simulink model "elevator"  (R2020a)
settings: Solver=VariableStepAuto  StartTime=0.0  StopTime=inf  RelTol=1e-3
PreLoadFcn:
  | slplc.api.loadDataTypes;
undefined symbols (not defined in the file): BOOL, DINT, INT, slplc
libraries: simulink x1
(part 30 of 38)

== system elevator/PLCControllerSuite/__Logic/Task/Program/__Logic/EQU/RungInOverride/ForceRungInFalseRead/__CoreLabelRead ==
  DataRead : DataStoreRead  DataStoreName=x_PLCLabel__s4_3653__Force_RungIn_False
  Out1 : Outport  VectorParamsAs1DForOutWhenUnconnected=off
  wires:
  DataRead/1 -> Out1/1

== system elevator/PLCControllerSuite/__Logic/Task/Program/__Logic/EQU1/RungInOverride/ForceRungInFalseRead/__CoreLabelRead ==
  DataRead : DataStoreRead  DataStoreName=x_PLCLabel__s4_3653__Force_RungIn_False
  Out1 : Outport  VectorParamsAs1DForOutWhenUnconnected=off
  wires:
  DataRead/1 -> Out1/1

== system elevator/PLCControllerSuite/__Logic/Task/Program/__Logic/EQU2/RungInOverride/ForceRungInFalseRead/__CoreLabelRead ==
  DataRead : DataStoreRead  DataStoreName=x_PLCLabel__s4_3653__Force_RungIn_False
  Out1 : Outport  VectorParamsAs1DForOutWhenUnconnected=off
  wires:
  DataRead/1 -> Out1/1

== system elevator/PLCControllerSuite/__Logic/Task/Program/__Logic/EQU3/RungInOverride/ForceRungInFalseRead/__CoreLabelRead ==
  DataRead : DataStoreRead  DataStoreName=x_PLCLabel__s4_3653__Force_RungIn_False
  Out1 : Outport  VectorParamsAs1DForOutWhenUnconnected=off
  wires:
  DataRead/1 -> Out1/1

== system elevator/PLCControllerSuite/__Logic/Task/Program/__Logic/GRT/RungInOverride/ForceRungInFalseRead/__CoreLabelRead ==
  DataRead : DataStoreRead  DataStoreName=x_PLCLabel__s4_3653__Force_RungIn_False
  Out1 : Outport  VectorParamsAs1DForOutWhenUnconnected=off
  wires:
  DataRead/1 -> Out1/1

== system elevator/PLCControllerSuite/__Logic/Task/Program/__Logic/LEQ/RungInOverride/ForceRungInFalseRead/__CoreLabelRead ==
  DataRead : DataStoreRead  DataStoreName=x_PLCLabel__s4_3653__Force_RungIn_False
  Out1 : Outport  VectorParamsAs1DForOutWhenUnconnected=off
  wires:
  DataRead/1 -> Out1/1

== system elevator/PLCControllerSuite/__Logic/Task/Program/__Logic/MOV/RungInOverride/ForceRungInFalseRead/__CoreLabelRead ==
  DataRead : DataStoreRead  DataStoreName=x_PLCLabel__s4_3653__Force_RungIn_False
  Out1 : Outport  VectorParamsAs1DForOutWhenUnconnected=off
  wires:
  DataRead/1 -> Out1/1

== system elevator/PLCControllerSuite/__Logic/Task/Program/__Logic/MOV/RungOutOverride/BlockEnableRead/__CoreLabelRead ==
  DataRead : DataStoreRead  DataStoreName=x_PLCLabel__s4_3653__Block_Enable
  Out1 : Outport  VectorParamsAs1DForOutWhenUnconnected=off
  wires:
  DataRead/1 -> Out1/1

== system elevator/PLCControllerSuite/__Logic/Task/Program/__Logic/MOV/RungOutOverride/VariableWriteEnableWrite/__CoreLabelWrite ==
  In1 : Inport
  DataWrite : DataStoreWrite  DataStoreName=x_PLCLabel__s4_3653__Variable_Write_Enable
  wires:
  In1/1 -> DataWrite/1

== system elevator/PLCControllerSuite/__Logic/Task/Program/__Logic/MOV1/RungInOverride/ForceRungInFalseRead/__CoreLabelRead ==
  DataRead : DataStoreRead  DataStoreName=x_PLCLabel__s4_3653__Force_RungIn_False
  Out1 : Outport  VectorParamsAs1DForOutWhenUnconnected=off
  wires:
  DataRead/1 -> Out1/1

== system elevator/PLCControllerSuite/__Logic/Task/Program/__Logic/MOV1/RungOutOverride/BlockEnableRead/__CoreLabelRead ==
  DataRead : DataStoreRead  DataStoreName=x_PLCLabel__s4_3653__Block_Enable
  Out1 : Outport  VectorParamsAs1DForOutWhenUnconnected=off
  wires:
  DataRead/1 -> Out1/1

== system elevator/PLCControllerSuite/__Logic/Task/Program/__Logic/MOV1/RungOutOverride/VariableWriteEnableWrite/__CoreLabelWrite ==
  In1 : Inport
  DataWrite : DataStoreWrite  DataStoreName=x_PLCLabel__s4_3653__Variable_Write_Enable
  wires:
  In1/1 -> DataWrite/1

== system elevator/PLCControllerSuite/__Logic/Task/Program/__Logic/MOV2/RungInOverride/ForceRungInFalseRead/__CoreLabelRead ==
  DataRead : DataStoreRead  DataStoreName=x_PLCLabel__s4_3653__Force_RungIn_False
  Out1 : Outport  VectorParamsAs1DForOutWhenUnconnected=off
  wires:
  DataRead/1 -> Out1/1

== system elevator/PLCControllerSuite/__Logic/Task/Program/__Logic/MOV2/RungOutOverride/BlockEnableRead/__CoreLabelRead ==
  DataRead : DataStoreRead  DataStoreName=x_PLCLabel__s4_3653__Block_Enable
  Out1 : Outport  VectorParamsAs1DForOutWhenUnconnected=off
  wires:
  DataRead/1 -> Out1/1

== system elevator/PLCControllerSuite/__Logic/Task/Program/__Logic/MOV2/RungOutOverride/VariableWriteEnableWrite/__CoreLabelWrite ==
  In1 : Inport
  DataWrite : DataStoreWrite  DataStoreName=x_PLCLabel__s4_3653__Variable_Write_Enable
  wires:
  In1/1 -> DataWrite/1

== system elevator/PLCControllerSuite/__Logic/Task/Program/__Logic/MOV3/RungInOverride/ForceRungInFalseRead/__CoreLabelRead ==
  DataRead : DataStoreRead  DataStoreName=x_PLCLabel__s4_3653__Force_RungIn_False
  Out1 : Outport  VectorParamsAs1DForOutWhenUnconnected=off
  wires:
  DataRead/1 -> Out1/1

== system elevator/PLCControllerSuite/__Logic/Task/Program/__Logic/MOV3/RungOutOverride/BlockEnableRead/__CoreLabelRead ==
  DataRead : DataStoreRead  DataStoreName=x_PLCLabel__s4_3653__Block_Enable
  Out1 : Outport  VectorParamsAs1DForOutWhenUnconnected=off
  wires:
  DataRead/1 -> Out1/1

== system elevator/PLCControllerSuite/__Logic/Task/Program/__Logic/MOV3/RungOutOverride/VariableWriteEnableWrite/__CoreLabelWrite ==
  In1 : Inport
  DataWrite : DataStoreWrite  DataStoreName=x_PLCLabel__s4_3653__Variable_Write_Enable
  wires:
  In1/1 -> DataWrite/1

== system elevator/PLCControllerSuite/__Logic/Task/Program/__Logic/MOV4/RungInOverride/ForceRungInFalseRead/__CoreLabelRead ==
  DataRead : DataStoreRead  DataStoreName=x_PLCLabel__s4_3653__Force_RungIn_False
  Out1 : Outport  VectorParamsAs1DForOutWhenUnconnected=off
  wires:
  DataRead/1 -> Out1/1

== system elevator/PLCControllerSuite/__Logic/Task/Program/__Logic/MOV4/RungOutOverride/BlockEnableRead/__CoreLabelRead ==
  DataRead : DataStoreRead  DataStoreName=x_PLCLabel__s4_3653__Block_Enable
  Out1 : Outport  VectorParamsAs1DForOutWhenUnconnected=off
  wires:
  DataRead/1 -> Out1/1

== system elevator/PLCControllerSuite/__Logic/Task/Program/__Logic/MOV4/RungOutOverride/VariableWriteEnableWrite/__CoreLabelWrite ==
  In1 : Inport
  DataWrite : DataStoreWrite  DataStoreName=x_PLCLabel__s4_3653__Variable_Write_Enable
  wires:
  In1/1 -> DataWrite/1

== system elevator/PLCControllerSuite/__Logic/Task/Program/__Logic/MUL/RungInOverride/ForceRungInFalseRead/__CoreLabelRead ==
  DataRead : DataStoreRead  DataStoreName=x_PLCLabel__s4_3653__Force_RungIn_False
  Out1 : Outport  VectorParamsAs1DForOutWhenUnconnected=off
  wires:
  DataRead/1 -> Out1/1

== system elevator/PLCControllerSuite/__Logic/Task/Program/__Logic/MUL/RungOutOverride/BlockEnableRead/__CoreLabelRead ==
  DataRead : DataStoreRead  DataStoreName=x_PLCLabel__s4_3653__Block_Enable
  Out1 : Outport  VectorParamsAs1DForOutWhenUnconnected=off
  wires:
  DataRead/1 -> Out1/1

== system elevator/PLCControllerSuite/__Logic/Task/Program/__Logic/MUL/RungOutOverride/VariableWriteEnableWrite/__CoreLabelWrite ==
  In1 : Inport
  DataWrite : DataStoreWrite  DataStoreName=x_PLCLabel__s4_3653__Variable_Write_Enable
  wires:
  In1/1 -> DataWrite/1

== system elevator/PLCControllerSuite/__Logic/Task/Program/__Logic/OTE/Instruction_Enable/Initialize Function/__CoreVarWrite ==
  u : Inport
  DataWrite : DataStoreWrite  DataStoreName=xxx_PLC_VAR_StartHold
  wires:
  u/1 -> DataWrite/1

== system elevator/PLCControllerSuite/__Logic/Task/Program/__Logic/OTE/Instruction_Enable/Rung-condition is false/__CoreVarWrite ==
  u : Inport
  DataWrite : DataStoreWrite  DataStoreName=xxx_PLC_VAR_StartHold
  wires:
  u/1 -> DataWrite/1

== system elevator/PLCControllerSuite/__Logic/Task/Program/__Logic/OTE/Instruction_Enable/Rung-condition-in is true/__CoreVarWrite ==
  u : Inport
  DataWrite : DataStoreWrite  DataStoreName=xxx_PLC_VAR_StartHold
  wires:
  u/1 -> DataWrite/1

== system elevator/PLCControllerSuite/__Logic/Task/Program/__Logic/OTE/RungInOverride/ForceRungInFalseRead/__CoreLabelRead ==
  DataRead : DataStoreRead  DataStoreName=x_PLCLabel__s4_3653__Force_RungIn_False
  Out1 : Outport  VectorParamsAs1DForOutWhenUnconnected=off
  wires:
  DataRead/1 -> Out1/1

== system elevator/PLCControllerSuite/__Logic/Task/Program/__Logic/OTE1/Instruction_Enable/Initialize Function/__CoreVarWrite ==
  u : Inport
  DataWrite : DataStoreWrite  DataStoreName=xxx_PLC_VAR_F1PBHold
  wires:
  u/1 -> DataWrite/1

== system elevator/PLCControllerSuite/__Logic/Task/Program/__Logic/OTE1/Instruction_Enable/Rung-condition is false/__CoreVarWrite ==
  u : Inport
  DataWrite : DataStoreWrite  DataStoreName=xxx_PLC_VAR_F1PBHold
  wires:
  u/1 -> DataWrite/1

== system elevator/PLCControllerSuite/__Logic/Task/Program/__Logic/OTE1/Instruction_Enable/Rung-condition-in is true/__CoreVarWrite ==
  u : Inport
  DataWrite : DataStoreWrite  DataStoreName=xxx_PLC_VAR_F1PBHold
  wires:
  u/1 -> DataWrite/1

== system elevator/PLCControllerSuite/__Logic/Task/Program/__Logic/OTE1/RungInOverride/ForceRungInFalseRead/__CoreLabelRead ==
  DataRead : DataStoreRead  DataStoreName=x_PLCLabel__s4_3653__Force_RungIn_False
  Out1 : Outport  VectorParamsAs1DForOutWhenUnconnected=off
  wires:
  DataRead/1 -> Out1/1

== system elevator/PLCControllerSuite/__Logic/Task/Program/__Logic/OTE10/Instruction_Enable/Initialize Function/__CoreVarWrite ==
  u : Inport
  DataWrite : DataStoreWrite  DataStoreName=xxx_PLC_VAR_MemoryGoDown
  wires:
  u/1 -> DataWrite/1

== system elevator/PLCControllerSuite/__Logic/Task/Program/__Logic/OTE10/Instruction_Enable/Rung-condition is false/__CoreVarWrite ==
  u : Inport
  DataWrite : DataStoreWrite  DataStoreName=xxx_PLC_VAR_MemoryGoDown
  wires:
  u/1 -> DataWrite/1

== system elevator/PLCControllerSuite/__Logic/Task/Program/__Logic/OTE10/Instruction_Enable/Rung-condition-in is true/__CoreVarWrite ==
  u : Inport
  DataWrite : DataStoreWrite  DataStoreName=xxx_PLC_VAR_MemoryGoDown
  wires:
  u/1 -> DataWrite/1

== system elevator/PLCControllerSuite/__Logic/Task/Program/__Logic/OTE10/RungInOverride/ForceRungInFalseRead/__CoreLabelRead ==
  DataRead : DataStoreRead  DataStoreName=x_PLCLabel__s4_3653__Force_RungIn_False
  Out1 : Outport  VectorParamsAs1DForOutWhenUnconnected=off
  wires:
  DataRead/1 -> Out1/1

== system elevator/PLCControllerSuite/__Logic/Task/Program/__Logic/OTE11/Instruction_Enable/Initialize Function/__CoreVarWrite ==
  u : Inport
  DataWrite : DataStoreWrite  DataStoreName=xxx_PLC_VAR_RMPUPTRG
  wires:
  u/1 -> DataWrite/1

== system elevator/PLCControllerSuite/__Logic/Task/Program/__Logic/OTE11/Instruction_Enable/Rung-condition is false/__CoreVarWrite ==
  u : Inport
  DataWrite : DataStoreWrite  DataStoreName=xxx_PLC_VAR_RMPUPTRG
  wires:
  u/1 -> DataWrite/1

== system elevator/PLCControllerSuite/__Logic/Task/Program/__Logic/OTE11/Instruction_Enable/Rung-condition-in is true/__CoreVarWrite ==
  u : Inport
  DataWrite : DataStoreWrite  DataStoreName=xxx_PLC_VAR_RMPUPTRG
  wires:
  u/1 -> DataWrite/1

== system elevator/PLCControllerSuite/__Logic/Task/Program/__Logic/OTE11/RungInOverride/ForceRungInFalseRead/__CoreLabelRead ==
  DataRead : DataStoreRead  DataStoreName=x_PLCLabel__s4_3653__Force_RungIn_False
  Out1 : Outport  VectorParamsAs1DForOutWhenUnconnected=off
  wires:
  DataRead/1 -> Out1/1

== system elevator/PLCControllerSuite/__Logic/Task/Program/__Logic/OTE12/Instruction_Enable/Initialize Function/__CoreVarWrite ==
  u : Inport
  DataWrite : DataStoreWrite  DataStoreName=xxx_PLC_VAR_RMPUP
  wires:
  u/1 -> DataWrite/1

== system elevator/PLCControllerSuite/__Logic/Task/Program/__Logic/OTE12/Instruction_Enable/Rung-condition is false/__CoreVarWrite ==
  u : Inport
  DataWrite : DataStoreWrite  DataStoreName=xxx_PLC_VAR_RMPUP
  wires:
  u/1 -> DataWrite/1

== system elevator/PLCControllerSuite/__Logic/Task/Program/__Logic/OTE12/Instruction_Enable/Rung-condition-in is true/__CoreVarWrite ==
  u : Inport
  DataWrite : DataStoreWrite  DataStoreName=xxx_PLC_VAR_RMPUP
  wires:
  u/1 -> DataWrite/1

== system elevator/PLCControllerSuite/__Logic/Task/Program/__Logic/OTE12/RungInOverride/ForceRungInFalseRead/__CoreLabelRead ==
  DataRead : DataStoreRead  DataStoreName=x_PLCLabel__s4_3653__Force_RungIn_False
  Out1 : Outport  VectorParamsAs1DForOutWhenUnconnected=off
  wires:
  DataRead/1 -> Out1/1

== system elevator/PLCControllerSuite/__Logic/Task/Program/__Logic/OTE13/Instruction_Enable/Initialize Function/__CoreVarWrite ==
  u : Inport
  DataWrite : DataStoreWrite  DataStoreName=xxx_PLC_VAR_RMPDN
  wires:
  u/1 -> DataWrite/1

== system elevator/PLCControllerSuite/__Logic/Task/Program/__Logic/OTE13/Instruction_Enable/Rung-condition is false/__CoreVarWrite ==
  u : Inport
  DataWrite : DataStoreWrite  DataStoreName=xxx_PLC_VAR_RMPDN
  wires:
  u/1 -> DataWrite/1

== system elevator/PLCControllerSuite/__Logic/Task/Program/__Logic/OTE13/Instruction_Enable/Rung-condition-in is true/__CoreVarWrite ==
  u : Inport
  DataWrite : DataStoreWrite  DataStoreName=xxx_PLC_VAR_RMPDN
  wires:
  u/1 -> DataWrite/1

== system elevator/PLCControllerSuite/__Logic/Task/Program/__Logic/OTE13/RungInOverride/ForceRungInFalseRead/__CoreLabelRead ==
  DataRead : DataStoreRead  DataStoreName=x_PLCLabel__s4_3653__Force_RungIn_False
  Out1 : Outport  VectorParamsAs1DForOutWhenUnconnected=off
  wires:
  DataRead/1 -> Out1/1

== system elevator/PLCControllerSuite/__Logic/Task/Program/__Logic/OTE14/Instruction_Enable/Initialize Function/__CoreVarWrite ==
  u : Inport
  DataWrite : DataStoreWrite  DataStoreName=xxx_PLC_VAR_RMPUPKIL
  wires:
  u/1 -> DataWrite/1

== system elevator/PLCControllerSuite/__Logic/Task/Program/__Logic/OTE14/Instruction_Enable/Rung-condition is false/__CoreVarWrite ==
  u : Inport
  DataWrite : DataStoreWrite  DataStoreName=xxx_PLC_VAR_RMPUPKIL
  wires:
  u/1 -> DataWrite/1

== system elevator/PLCControllerSuite/__Logic/Task/Program/__Logic/OTE14/Instruction_Enable/Rung-condition-in is true/__CoreVarWrite ==
  u : Inport
  DataWrite : DataStoreWrite  DataStoreName=xxx_PLC_VAR_RMPUPKIL
  wires:
  u/1 -> DataWrite/1

== system elevator/PLCControllerSuite/__Logic/Task/Program/__Logic/OTE14/RungInOverride/ForceRungInFalseRead/__CoreLabelRead ==
  DataRead : DataStoreRead  DataStoreName=x_PLCLabel__s4_3653__Force_RungIn_False
  Out1 : Outport  VectorParamsAs1DForOutWhenUnconnected=off
  wires:
  DataRead/1 -> Out1/1

== system elevator/PLCControllerSuite/__Logic/Task/Program/__Logic/OTE15/Instruction_Enable/Initialize Function/__CoreVarWrite ==
  u : Inport
  DataWrite : DataStoreWrite  DataStoreName=xxx_PLC_VAR_TempS1HUp
  wires:
  u/1 -> DataWrite/1

== system elevator/PLCControllerSuite/__Logic/Task/Program/__Logic/OTE15/Instruction_Enable/Rung-condition is false/__CoreVarWrite ==
  u : Inport
  DataWrite : DataStoreWrite  DataStoreName=xxx_PLC_VAR_TempS1HUp
  wires:
  u/1 -> DataWrite/1

== system elevator/PLCControllerSuite/__Logic/Task/Program/__Logic/OTE15/Instruction_Enable/Rung-condition-in is true/__CoreVarWrite ==
  u : Inport
  DataWrite : DataStoreWrite  DataStoreName=xxx_PLC_VAR_TempS1HUp
  wires:
  u/1 -> DataWrite/1

== system elevator/PLCControllerSuite/__Logic/Task/Program/__Logic/OTE15/RungInOverride/ForceRungInFalseRead/__CoreLabelRead ==
  DataRead : DataStoreRead  DataStoreName=x_PLCLabel__s4_3653__Force_RungIn_False
  Out1 : Outport  VectorParamsAs1DForOutWhenUnconnected=off
  wires:
  DataRead/1 -> Out1/1

== system elevator/PLCControllerSuite/__Logic/Task/Program/__Logic/OTE16/Instruction_Enable/Initialize Function/__CoreVarWrite ==
  u : Inport
  DataWrite : DataStoreWrite  DataStoreName=xxx_PLC_VAR_TempS2LUp
  wires:
  u/1 -> DataWrite/1

== system elevator/PLCControllerSuite/__Logic/Task/Program/__Logic/OTE16/Instruction_Enable/Rung-condition is false/__CoreVarWrite ==
  u : Inport
  DataWrite : DataStoreWrite  DataStoreName=xxx_PLC_VAR_TempS2LUp
  wires:
  u/1 -> DataWrite/1

== system elevator/PLCControllerSuite/__Logic/Task/Program/__Logic/OTE16/Instruction_Enable/Rung-condition-in is true/__CoreVarWrite ==
  u : Inport
  DataWrite : DataStoreWrite  DataStoreName=xxx_PLC_VAR_TempS2LUp
  wires:
  u/1 -> DataWrite/1

== system elevator/PLCControllerSuite/__Logic/Task/Program/__Logic/OTE16/RungInOverride/ForceRungInFalseRead/__CoreLabelRead ==
  DataRead : DataStoreRead  DataStoreName=x_PLCLabel__s4_3653__Force_RungIn_False
  Out1 : Outport  VectorParamsAs1DForOutWhenUnconnected=off
  wires:
  DataRead/1 -> Out1/1

== system elevator/PLCControllerSuite/__Logic/Task/Program/__Logic/OTE17/Instruction_Enable/Initialize Function/__CoreVarWrite ==
  u : Inport
  DataWrite : DataStoreWrite  DataStoreName=xxx_PLC_VAR_TempS3LUp
  wires:
  u/1 -> DataWrite/1

== system elevator/PLCControllerSuite/__Logic/Task/Program/__Logic/OTE17/Instruction_Enable/Rung-condition is false/__CoreVarWrite ==
  u : Inport
  DataWrite : DataStoreWrite  DataStoreName=xxx_PLC_VAR_TempS3LUp
  wires:
  u/1 -> DataWrite/1

== system elevator/PLCControllerSuite/__Logic/Task/Program/__Logic/OTE17/Instruction_Enable/Rung-condition-in is true/__CoreVarWrite ==
  u : Inport
  DataWrite : DataStoreWrite  DataStoreName=xxx_PLC_VAR_TempS3LUp
  wires:
  u/1 -> DataWrite/1

== system elevator/PLCControllerSuite/__Logic/Task/Program/__Logic/OTE17/RungInOverride/ForceRungInFalseRead/__CoreLabelRead ==
  DataRead : DataStoreRead  DataStoreName=x_PLCLabel__s4_3653__Force_RungIn_False
  Out1 : Outport  VectorParamsAs1DForOutWhenUnconnected=off
  wires:
  DataRead/1 -> Out1/1

== system elevator/PLCControllerSuite/__Logic/Task/Program/__Logic/OTE18/Instruction_Enable/Initialize Function/__CoreVarWrite ==
  u : Inport
  DataWrite : DataStoreWrite  DataStoreName=xxx_PLC_VAR_TempS2HDown
  wires:
  u/1 -> DataWrite/1

== system elevator/PLCControllerSuite/__Logic/Task/Program/__Logic/OTE18/Instruction_Enable/Rung-condition is false/__CoreVarWrite ==
  u : Inport
  DataWrite : DataStoreWrite  DataStoreName=xxx_PLC_VAR_TempS2HDown
  wires:
  u/1 -> DataWrite/1

== system elevator/PLCControllerSuite/__Logic/Task/Program/__Logic/OTE18/Instruction_Enable/Rung-condition-in is true/__CoreVarWrite ==
  u : Inport
  DataWrite : DataStoreWrite  DataStoreName=xxx_PLC_VAR_TempS2HDown
  wires:
  u/1 -> DataWrite/1

== system elevator/PLCControllerSuite/__Logic/Task/Program/__Logic/OTE18/RungInOverride/ForceRungInFalseRead/__CoreLabelRead ==
  DataRead : DataStoreRead  DataStoreName=x_PLCLabel__s4_3653__Force_RungIn_False
  Out1 : Outport  VectorParamsAs1DForOutWhenUnconnected=off
  wires:
  DataRead/1 -> Out1/1

== system elevator/PLCControllerSuite/__Logic/Task/Program/__Logic/OTE19/Instruction_Enable/Initialize Function/__CoreVarWrite ==
  u : Inport
  DataWrite : DataStoreWrite  DataStoreName=xxx_PLC_VAR_TempS2LDown
  wires:
  u/1 -> DataWrite/1

== system elevator/PLCControllerSuite/__Logic/Task/Program/__Logic/OTE19/Instruction_Enable/Rung-condition is false/__CoreVarWrite ==
  u : Inport
  DataWrite : DataStoreWrite  DataStoreName=xxx_PLC_VAR_TempS2LDown
  wires:
  u/1 -> DataWrite/1

== system elevator/PLCControllerSuite/__Logic/Task/Program/__Logic/OTE19/Instruction_Enable/Rung-condition-in is true/__CoreVarWrite ==
  u : Inport
  DataWrite : DataStoreWrite  DataStoreName=xxx_PLC_VAR_TempS2LDown
  wires:
  u/1 -> DataWrite/1

== system elevator/PLCControllerSuite/__Logic/Task/Program/__Logic/OTE19/RungInOverride/ForceRungInFalseRead/__CoreLabelRead ==
  DataRead : DataStoreRead  DataStoreName=x_PLCLabel__s4_3653__Force_RungIn_False
  Out1 : Outport  VectorParamsAs1DForOutWhenUnconnected=off
  wires:
  DataRead/1 -> Out1/1

== system elevator/PLCControllerSuite/__Logic/Task/Program/__Logic/OTE2/Instruction_Enable/Initialize Function/__CoreVarWrite ==
  u : Inport
  DataWrite : DataStoreWrite  DataStoreName=xxx_PLC_VAR_F2PBHold
  wires:
  u/1 -> DataWrite/1

== system elevator/PLCControllerSuite/__Logic/Task/Program/__Logic/OTE2/Instruction_Enable/Rung-condition is false/__CoreVarWrite ==
  u : Inport
  DataWrite : DataStoreWrite  DataStoreName=xxx_PLC_VAR_F2PBHold
  wires:
  u/1 -> DataWrite/1

== system elevator/PLCControllerSuite/__Logic/Task/Program/__Logic/OTE2/Instruction_Enable/Rung-condition-in is true/__CoreVarWrite ==
  u : Inport
  DataWrite : DataStoreWrite  DataStoreName=xxx_PLC_VAR_F2PBHold
  wires:
  u/1 -> DataWrite/1

== system elevator/PLCControllerSuite/__Logic/Task/Program/__Logic/OTE2/RungInOverride/ForceRungInFalseRead/__CoreLabelRead ==
  DataRead : DataStoreRead  DataStoreName=x_PLCLabel__s4_3653__Force_RungIn_False
  Out1 : Outport  VectorParamsAs1DForOutWhenUnconnected=off
  wires:
  DataRead/1 -> Out1/1

== system elevator/PLCControllerSuite/__Logic/Task/Program/__Logic/OTE20/Instruction_Enable/Initialize Function/__CoreVarWrite ==
  u : Inport
  DataWrite : DataStoreWrite  DataStoreName=xxx_PLC_VAR_TempS1HDown
  wires:
  u/1 -> DataWrite/1

== system elevator/PLCControllerSuite/__Logic/Task/Program/__Logic/OTE20/Instruction_Enable/Rung-condition is false/__CoreVarWrite ==
  u : Inport
  DataWrite : DataStoreWrite  DataStoreName=xxx_PLC_VAR_TempS1HDown
  wires:
  u/1 -> DataWrite/1

== system elevator/PLCControllerSuite/__Logic/Task/Program/__Logic/OTE20/Instruction_Enable/Rung-condition-in is true/__CoreVarWrite ==
  u : Inport
  DataWrite : DataStoreWrite  DataStoreName=xxx_PLC_VAR_TempS1HDown
  wires:
  u/1 -> DataWrite/1

== system elevator/PLCControllerSuite/__Logic/Task/Program/__Logic/OTE20/RungInOverride/ForceRungInFalseRead/__CoreLabelRead ==
  DataRead : DataStoreRead  DataStoreName=x_PLCLabel__s4_3653__Force_RungIn_False
  Out1 : Outport  VectorParamsAs1DForOutWhenUnconnected=off
  wires:
  DataRead/1 -> Out1/1

== system elevator/PLCControllerSuite/__Logic/Task/Program/__Logic/OTE21/Instruction_Enable/Initialize Function/__CoreVarWrite ==
  u : Inport
  DataWrite : DataStoreWrite  DataStoreName=xxx_PLC_VAR_TempS2HUp
  wires:
  u/1 -> DataWrite/1

== system elevator/PLCControllerSuite/__Logic/Task/Program/__Logic/OTE21/Instruction_Enable/Rung-condition is false/__CoreVarWrite ==
  u : Inport
  DataWrite : DataStoreWrite  DataStoreName=xxx_PLC_VAR_TempS2HUp
  wires:
  u/1 -> DataWrite/1

== system elevator/PLCControllerSuite/__Logic/Task/Program/__Logic/OTE21/Instruction_Enable/Rung-condition-in is true/__CoreVarWrite ==
  u : Inport
  DataWrite : DataStoreWrite  DataStoreName=xxx_PLC_VAR_TempS2HUp
  wires:
  u/1 -> DataWrite/1

== system elevator/PLCControllerSuite/__Logic/Task/Program/__Logic/OTE21/RungInOverride/ForceRungInFalseRead/__CoreLabelRead ==
  DataRead : DataStoreRead  DataStoreName=x_PLCLabel__s4_3653__Force_RungIn_False
  Out1 : Outport  VectorParamsAs1DForOutWhenUnconnected=off
  wires:
  DataRead/1 -> Out1/1

== system elevator/PLCControllerSuite/__Logic/Task/Program/__Logic/OTE22/Instruction_Enable/Initialize Function/__CoreVarWrite ==
  u : Inport
  DataWrite : DataStoreWrite  DataStoreName=xxx_PLC_VAR_TempS3LDown
  wires:
  u/1 -> DataWrite/1

== system elevator/PLCControllerSuite/__Logic/Task/Program/__Logic/OTE22/Instruction_Enable/Rung-condition is false/__CoreVarWrite ==
  u : Inport
  DataWrite : DataStoreWrite  DataStoreName=xxx_PLC_VAR_TempS3LDown
  wires:
  u/1 -> DataWrite/1

== system elevator/PLCControllerSuite/__Logic/Task/Program/__Logic/OTE22/Instruction_Enable/Rung-condition-in is true/__CoreVarWrite ==
  u : Inport
  DataWrite : DataStoreWrite  DataStoreName=xxx_PLC_VAR_TempS3LDown
  wires:
  u/1 -> DataWrite/1

== system elevator/PLCControllerSuite/__Logic/Task/Program/__Logic/OTE22/RungInOverride/ForceRungInFalseRead/__CoreLabelRead ==
  DataRead : DataStoreRead  DataStoreName=x_PLCLabel__s4_3653__Force_RungIn_False
  Out1 : Outport  VectorParamsAs1DForOutWhenUnconnected=off
  wires:
  DataRead/1 -> Out1/1

== system elevator/PLCControllerSuite/__Logic/Task/Program/__Logic/OTE23/Instruction_Enable/Initialize Function/__CoreVarWrite ==
  u : Inport
  DataWrite : DataStoreWrite  DataStoreName=xxx_PLC_VAR_AtFloor1
  wires:
  u/1 -> DataWrite/1

== system elevator/PLCControllerSuite/__Logic/Task/Program/__Logic/OTE23/Instruction_Enable/Rung-condition is false/__CoreVarWrite ==
  u : Inport
  DataWrite : DataStoreWrite  DataStoreName=xxx_PLC_VAR_AtFloor1
  wires:
  u/1 -> DataWrite/1

== system elevator/PLCControllerSuite/__Logic/Task/Program/__Logic/OTE23/Instruction_Enable/Rung-condition-in is true/__CoreVarWrite ==
  u : Inport
  DataWrite : DataStoreWrite  DataStoreName=xxx_PLC_VAR_AtFloor1
  wires:
  u/1 -> DataWrite/1

== system elevator/PLCControllerSuite/__Logic/Task/Program/__Logic/OTE23/RungInOverride/ForceRungInFalseRead/__CoreLabelRead ==
  DataRead : DataStoreRead  DataStoreName=x_PLCLabel__s4_3653__Force_RungIn_False
  Out1 : Outport  VectorParamsAs1DForOutWhenUnconnected=off
  wires:
  DataRead/1 -> Out1/1

== system elevator/PLCControllerSuite/__Logic/Task/Program/__Logic/OTE24/Instruction_Enable/Initialize Function/__CoreVarWrite ==
  u : Inport
  DataWrite : DataStoreWrite  DataStoreName=xxx_PLC_VAR_AtFloor2
  wires:
  u/1 -> DataWrite/1

== system elevator/PLCControllerSuite/__Logic/Task/Program/__Logic/OTE24/Instruction_Enable/Rung-condition is false/__CoreVarWrite ==
  u : Inport
  DataWrite : DataStoreWrite  DataStoreName=xxx_PLC_VAR_AtFloor2
  wires:
  u/1 -> DataWrite/1

== system elevator/PLCControllerSuite/__Logic/Task/Program/__Logic/OTE24/Instruction_Enable/Rung-condition-in is true/__CoreVarWrite ==
  u : Inport
  DataWrite : DataStoreWrite  DataStoreName=xxx_PLC_VAR_AtFloor2
  wires:
  u/1 -> DataWrite/1

== system elevator/PLCControllerSuite/__Logic/Task/Program/__Logic/OTE24/RungInOverride/ForceRungInFalseRead/__CoreLabelRead ==
  DataRead : DataStoreRead  DataStoreName=x_PLCLabel__s4_3653__Force_RungIn_False
  Out1 : Outport  VectorParamsAs1DForOutWhenUnconnected=off
  wires:
  DataRead/1 -> Out1/1

== system elevator/PLCControllerSuite/__Logic/Task/Program/__Logic/OTE25/Instruction_Enable/Initialize Function/__CoreVarWrite ==
  u : Inport
  DataWrite : DataStoreWrite  DataStoreName=xxx_PLC_VAR_AtFloor3
  wires:
  u/1 -> DataWrite/1

== system elevator/PLCControllerSuite/__Logic/Task/Program/__Logic/OTE25/Instruction_Enable/Rung-condition is false/__CoreVarWrite ==
  u : Inport
  DataWrite : DataStoreWrite  DataStoreName=xxx_PLC_VAR_AtFloor3
  wires:
  u/1 -> DataWrite/1

== system elevator/PLCControllerSuite/__Logic/Task/Program/__Logic/OTE25/Instruction_Enable/Rung-condition-in is true/__CoreVarWrite ==
  u : Inport
  DataWrite : DataStoreWrite  DataStoreName=xxx_PLC_VAR_AtFloor3
  wires:
  u/1 -> DataWrite/1

== system elevator/PLCControllerSuite/__Logic/Task/Program/__Logic/OTE25/RungInOverride/ForceRungInFalseRead/__CoreLabelRead ==
  DataRead : DataStoreRead  DataStoreName=x_PLCLabel__s4_3653__Force_RungIn_False
  Out1 : Outport  VectorParamsAs1DForOutWhenUnconnected=off
  wires:
  DataRead/1 -> Out1/1

== system elevator/PLCControllerSuite/__Logic/Task/Program/__Logic/OTE26/Instruction_Enable/Initialize Function/__CoreVarWrite ==
  u : Inport
  DataWrite : DataStoreWrite  DataStoreName=xxx_PLC_VAR_GOINGUP
  wires:
  u/1 -> DataWrite/1

== system elevator/PLCControllerSuite/__Logic/Task/Program/__Logic/OTE26/Instruction_Enable/Rung-condition is false/__CoreVarWrite ==
  u : Inport
  DataWrite : DataStoreWrite  DataStoreName=xxx_PLC_VAR_GOINGUP
  wires:
  u/1 -> DataWrite/1

== system elevator/PLCControllerSuite/__Logic/Task/Program/__Logic/OTE26/Instruction_Enable/Rung-condition-in is true/__CoreVarWrite ==
  u : Inport
  DataWrite : DataStoreWrite  DataStoreName=xxx_PLC_VAR_GOINGUP
  wires:
  u/1 -> DataWrite/1

== system elevator/PLCControllerSuite/__Logic/Task/Program/__Logic/OTE26/RungInOverride/ForceRungInFalseRead/__CoreLabelRead ==
  DataRead : DataStoreRead  DataStoreName=x_PLCLabel__s4_3653__Force_RungIn_False
  Out1 : Outport  VectorParamsAs1DForOutWhenUnconnected=off
  wires:
  DataRead/1 -> Out1/1

== system elevator/PLCControllerSuite/__Logic/Task/Program/__Logic/OTE27/Instruction_Enable/Initialize Function/__CoreVarWrite ==
  u : Inport
  DataWrite : DataStoreWrite  DataStoreName=xxx_PLC_VAR_GOINGDN
  wires:
  u/1 -> DataWrite/1

== system elevator/PLCControllerSuite/__Logic/Task/Program/__Logic/OTE27/Instruction_Enable/Rung-condition is false/__CoreVarWrite ==
  u : Inport
  DataWrite : DataStoreWrite  DataStoreName=xxx_PLC_VAR_GOINGDN
  wires:
  u/1 -> DataWrite/1

== system elevator/PLCControllerSuite/__Logic/Task/Program/__Logic/OTE27/Instruction_Enable/Rung-condition-in is true/__CoreVarWrite ==
  u : Inport
  DataWrite : DataStoreWrite  DataStoreName=xxx_PLC_VAR_GOINGDN
  wires:
  u/1 -> DataWrite/1

== system elevator/PLCControllerSuite/__Logic/Task/Program/__Logic/OTE27/RungInOverride/ForceRungInFalseRead/__CoreLabelRead ==
  DataRead : DataStoreRead  DataStoreName=x_PLCLabel__s4_3653__Force_RungIn_False
  Out1 : Outport  VectorParamsAs1DForOutWhenUnconnected=off
  wires:
  DataRead/1 -> Out1/1

== system elevator/PLCControllerSuite/__Logic/Task/Program/__Logic/OTE28/Instruction_Enable/Initialize Function/__CoreVarWrite ==
  u : Inport
  DataWrite : DataStoreWrite  DataStoreName=xxx_PLC_VAR_MTRON
  wires:
  u/1 -> DataWrite/1

== system elevator/PLCControllerSuite/__Logic/Task/Program/__Logic/OTE28/Instruction_Enable/Rung-condition is false/__CoreVarWrite ==
  u : Inport
  DataWrite : DataStoreWrite  DataStoreName=xxx_PLC_VAR_MTRON
  wires:
  u/1 -> DataWrite/1

== system elevator/PLCControllerSuite/__Logic/Task/Program/__Logic/OTE28/Instruction_Enable/Rung-condition-in is true/__CoreVarWrite ==
  u : Inport
  DataWrite : DataStoreWrite  DataStoreName=xxx_PLC_VAR_MTRON
  wires:
  u/1 -> DataWrite/1

== system elevator/PLCControllerSuite/__Logic/Task/Program/__Logic/OTE28/RungInOverride/ForceRungInFalseRead/__CoreLabelRead ==
  DataRead : DataStoreRead  DataStoreName=x_PLCLabel__s4_3653__Force_RungIn_False
  Out1 : Outport  VectorParamsAs1DForOutWhenUnconnected=off
  wires:
  DataRead/1 -> Out1/1

== system elevator/PLCControllerSuite/__Logic/Task/Program/__Logic/OTE29/Instruction_Enable/Initialize Function/__CoreVarWrite ==
  u : Inport
  DataWrite : DataStoreWrite  DataStoreName=xxx_PLC_VAR_RMPDNTRG
  wires:
  u/1 -> DataWrite/1

== system elevator/PLCControllerSuite/__Logic/Task/Program/__Logic/OTE29/Instruction_Enable/Rung-condition is false/__CoreVarWrite ==
  u : Inport
  DataWrite : DataStoreWrite  DataStoreName=xxx_PLC_VAR_RMPDNTRG
  wires:
  u/1 -> DataWrite/1

== system elevator/PLCControllerSuite/__Logic/Task/Program/__Logic/OTE29/Instruction_Enable/Rung-condition-in is true/__CoreVarWrite ==
  u : Inport
  DataWrite : DataStoreWrite  DataStoreName=xxx_PLC_VAR_RMPDNTRG
  wires:
  u/1 -> DataWrite/1

== system elevator/PLCControllerSuite/__Logic/Task/Program/__Logic/OTE29/RungInOverride/ForceRungInFalseRead/__CoreLabelRead ==
  DataRead : DataStoreRead  DataStoreName=x_PLCLabel__s4_3653__Force_RungIn_False
  Out1 : Outport  VectorParamsAs1DForOutWhenUnconnected=off
  wires:
  DataRead/1 -> Out1/1

== system elevator/PLCControllerSuite/__Logic/Task/Program/__Logic/OTE3/Instruction_Enable/Initialize Function/__CoreVarWrite ==
  u : Inport
  DataWrite : DataStoreWrite  DataStoreName=xxx_PLC_VAR_F3PBHold
  wires:
  u/1 -> DataWrite/1

== system elevator/PLCControllerSuite/__Logic/Task/Program/__Logic/OTE3/Instruction_Enable/Rung-condition is false/__CoreVarWrite ==
  u : Inport
  DataWrite : DataStoreWrite  DataStoreName=xxx_PLC_VAR_F3PBHold
  wires:
  u/1 -> DataWrite/1

== system elevator/PLCControllerSuite/__Logic/Task/Program/__Logic/OTE3/Instruction_Enable/Rung-condition-in is true/__CoreVarWrite ==
  u : Inport
  DataWrite : DataStoreWrite  DataStoreName=xxx_PLC_VAR_F3PBHold
  wires:
  u/1 -> DataWrite/1

== system elevator/PLCControllerSuite/__Logic/Task/Program/__Logic/OTE3/RungInOverride/ForceRungInFalseRead/__CoreLabelRead ==
  DataRead : DataStoreRead  DataStoreName=x_PLCLabel__s4_3653__Force_RungIn_False
  Out1 : Outport  VectorParamsAs1DForOutWhenUnconnected=off
  wires:
  DataRead/1 -> Out1/1

== system elevator/PLCControllerSuite/__Logic/Task/Program/__Logic/OTE30/Instruction_Enable/Initialize Function/__CoreVarWrite ==
  u : Inport
  DataWrite : DataStoreWrite  DataStoreName=xxx_PLC_VAR_INCSPD
  wires:
  u/1 -> DataWrite/1

== system elevator/PLCControllerSuite/__Logic/Task/Program/__Logic/OTE30/Instruction_Enable/Rung-condition is false/__CoreVarWrite ==
  u : Inport
  DataWrite : DataStoreWrite  DataStoreName=xxx_PLC_VAR_INCSPD
  wires:
  u/1 -> DataWrite/1

== system elevator/PLCControllerSuite/__Logic/Task/Program/__Logic/OTE30/Instruction_Enable/Rung-condition-in is true/__CoreVarWrite ==
  u : Inport
  DataWrite : DataStoreWrite  DataStoreName=xxx_PLC_VAR_INCSPD
  wires:
  u/1 -> DataWrite/1

== system elevator/PLCControllerSuite/__Logic/Task/Program/__Logic/OTE30/RungInOverride/ForceRungInFalseRead/__CoreLabelRead ==
  DataRead : DataStoreRead  DataStoreName=x_PLCLabel__s4_3653__Force_RungIn_False
  Out1 : Outport  VectorParamsAs1DForOutWhenUnconnected=off
  wires:
  DataRead/1 -> Out1/1

== system elevator/PLCControllerSuite/__Logic/Task/Program/__Logic/OTE31/Instruction_Enable/Initialize Function/__CoreVarWrite ==
  u : Inport
  DataWrite : DataStoreWrite  DataStoreName=xxx_PLC_VAR_DECSPD
  wires:
  u/1 -> DataWrite/1

== system elevator/PLCControllerSuite/__Logic/Task/Program/__Logic/OTE31/Instruction_Enable/Rung-condition is false/__CoreVarWrite ==
  u : Inport
  DataWrite : DataStoreWrite  DataStoreName=xxx_PLC_VAR_DECSPD
  wires:
  u/1 -> DataWrite/1

== system elevator/PLCControllerSuite/__Logic/Task/Program/__Logic/OTE31/Instruction_Enable/Rung-condition-in is true/__CoreVarWrite ==
  u : Inport
  DataWrite : DataStoreWrite  DataStoreName=xxx_PLC_VAR_DECSPD
  wires:
  u/1 -> DataWrite/1

== system elevator/PLCControllerSuite/__Logic/Task/Program/__Logic/OTE31/RungInOverride/ForceRungInFalseRead/__CoreLabelRead ==
  DataRead : DataStoreRead  DataStoreName=x_PLCLabel__s4_3653__Force_RungIn_False
  Out1 : Outport  VectorParamsAs1DForOutWhenUnconnected=off
  wires:
  DataRead/1 -> Out1/1

== system elevator/PLCControllerSuite/__Logic/Task/Program/__Logic/OTE4/Instruction_Enable/Initialize Function/__CoreVarWrite ==
  u : Inport
  DataWrite : DataStoreWrite  DataStoreName=xxx_PLC_VAR_F1UpBHold
  wires:
  u/1 -> DataWrite/1

== system elevator/PLCControllerSuite/__Logic/Task/Program/__Logic/OTE4/Instruction_Enable/Rung-condition is false/__CoreVarWrite ==
  u : Inport
  DataWrite : DataStoreWrite  DataStoreName=xxx_PLC_VAR_F1UpBHold
  wires:
  u/1 -> DataWrite/1

== system elevator/PLCControllerSuite/__Logic/Task/Program/__Logic/OTE4/Instruction_Enable/Rung-condition-in is true/__CoreVarWrite ==
  u : Inport
  DataWrite : DataStoreWrite  DataStoreName=xxx_PLC_VAR_F1UpBHold
  wires:
  u/1 -> DataWrite/1

== system elevator/PLCControllerSuite/__Logic/Task/Program/__Logic/OTE4/RungInOverride/ForceRungInFalseRead/__CoreLabelRead ==
  DataRead : DataStoreRead  DataStoreName=x_PLCLabel__s4_3653__Force_RungIn_False
  Out1 : Outport  VectorParamsAs1DForOutWhenUnconnected=off
  wires:
  DataRead/1 -> Out1/1

== system elevator/PLCControllerSuite/__Logic/Task/Program/__Logic/OTE5/Instruction_Enable/Initialize Function/__CoreVarWrite ==
  u : Inport
  DataWrite : DataStoreWrite  DataStoreName=xxx_PLC_VAR_F2UpDownBHold
  wires:
  u/1 -> DataWrite/1

== system elevator/PLCControllerSuite/__Logic/Task/Program/__Logic/OTE5/Instruction_Enable/Rung-condition is false/__CoreVarWrite ==
  u : Inport
  DataWrite : DataStoreWrite  DataStoreName=xxx_PLC_VAR_F2UpDownBHold
  wires:
  u/1 -> DataWrite/1

== system elevator/PLCControllerSuite/__Logic/Task/Program/__Logic/OTE5/Instruction_Enable/Rung-condition-in is true/__CoreVarWrite ==
  u : Inport
  DataWrite : DataStoreWrite  DataStoreName=xxx_PLC_VAR_F2UpDownBHold
  wires:
  u/1 -> DataWrite/1

== system elevator/PLCControllerSuite/__Logic/Task/Program/__Logic/OTE5/RungInOverride/ForceRungInFalseRead/__CoreLabelRead ==
  DataRead : DataStoreRead  DataStoreName=x_PLCLabel__s4_3653__Force_RungIn_False
  Out1 : Outport  VectorParamsAs1DForOutWhenUnconnected=off
  wires:
  DataRead/1 -> Out1/1

== system elevator/PLCControllerSuite/__Logic/Task/Program/__Logic/OTE6/Instruction_Enable/Initialize Function/__CoreVarWrite ==
  u : Inport
  DataWrite : DataStoreWrite  DataStoreName=xxx_PLC_VAR_F3DownBHold
  wires:
  u/1 -> DataWrite/1

== system elevator/PLCControllerSuite/__Logic/Task/Program/__Logic/OTE6/Instruction_Enable/Rung-condition is false/__CoreVarWrite ==
  u : Inport
  DataWrite : DataStoreWrite  DataStoreName=xxx_PLC_VAR_F3DownBHold
  wires:
  u/1 -> DataWrite/1

== system elevator/PLCControllerSuite/__Logic/Task/Program/__Logic/OTE6/Instruction_Enable/Rung-condition-in is true/__CoreVarWrite ==
  u : Inport
  DataWrite : DataStoreWrite  DataStoreName=xxx_PLC_VAR_F3DownBHold
  wires:
  u/1 -> DataWrite/1

== system elevator/PLCControllerSuite/__Logic/Task/Program/__Logic/OTE6/RungInOverride/ForceRungInFalseRead/__CoreLabelRead ==
  DataRead : DataStoreRead  DataStoreName=x_PLCLabel__s4_3653__Force_RungIn_False
  Out1 : Outport  VectorParamsAs1DForOutWhenUnconnected=off
  wires:
  DataRead/1 -> Out1/1

== system elevator/PLCControllerSuite/__Logic/Task/Program/__Logic/OTE7/Instruction_Enable/Initialize Function/__CoreVarWrite ==
  u : Inport
  DataWrite : DataStoreWrite  DataStoreName=xxx_PLC_VAR_SENCHK
  wires:
  u/1 -> DataWrite/1

== system elevator/PLCControllerSuite/__Logic/Task/Program/__Logic/OTE7/Instruction_Enable/Rung-condition is false/__CoreVarWrite ==
  u : Inport
  DataWrite : DataStoreWrite  DataStoreName=xxx_PLC_VAR_SENCHK
  wires:
  u/1 -> DataWrite/1

== system elevator/PLCControllerSuite/__Logic/Task/Program/__Logic/OTE7/Instruction_Enable/Rung-condition-in is true/__CoreVarWrite ==
  u : Inport
  DataWrite : DataStoreWrite  DataStoreName=xxx_PLC_VAR_SENCHK
  wires:
  u/1 -> DataWrite/1

== system elevator/PLCControllerSuite/__Logic/Task/Program/__Logic/OTE7/RungInOverride/ForceRungInFalseRead/__CoreLabelRead ==
  DataRead : DataStoreRead  DataStoreName=x_PLCLabel__s4_3653__Force_RungIn_False
  Out1 : Outport  VectorParamsAs1DForOutWhenUnconnected=off
  wires:
  DataRead/1 -> Out1/1

== system elevator/PLCControllerSuite/__Logic/Task/Program/__Logic/OTE8/Instruction_Enable/Initialize Function/__CoreVarWrite ==
  u : Inport
  DataWrite : DataStoreWrite  DataStoreName=xxx_PLC_VAR_LSTDIRUP
  wires:
  u/1 -> DataWrite/1

== system elevator/PLCControllerSuite/__Logic/Task/Program/__Logic/OTE8/Instruction_Enable/Rung-condition is false/__CoreVarWrite ==
  u : Inport
  DataWrite : DataStoreWrite  DataStoreName=xxx_PLC_VAR_LSTDIRUP
  wires:
  u/1 -> DataWrite/1

== system elevator/PLCControllerSuite/__Logic/Task/Program/__Logic/OTE8/Instruction_Enable/Rung-condition-in is true/__CoreVarWrite ==
  u : Inport
  DataWrite : DataStoreWrite  DataStoreName=xxx_PLC_VAR_LSTDIRUP
  wires:
  u/1 -> DataWrite/1

== system elevator/PLCControllerSuite/__Logic/Task/Program/__Logic/OTE8/RungInOverride/ForceRungInFalseRead/__CoreLabelRead ==
  DataRead : DataStoreRead  DataStoreName=x_PLCLabel__s4_3653__Force_RungIn_False
  Out1 : Outport  VectorParamsAs1DForOutWhenUnconnected=off
  wires:
  DataRead/1 -> Out1/1

== system elevator/PLCControllerSuite/__Logic/Task/Program/__Logic/OTE9/Instruction_Enable/Initialize Function/__CoreVarWrite ==
  u : Inport
  DataWrite : DataStoreWrite  DataStoreName=xxx_PLC_VAR_MemoryGoUp
  wires:
  u/1 -> DataWrite/1

== system elevator/PLCControllerSuite/__Logic/Task/Program/__Logic/OTE9/Instruction_Enable/Rung-condition is false/__CoreVarWrite ==
  u : Inport
  DataWrite : DataStoreWrite  DataStoreName=xxx_PLC_VAR_MemoryGoUp
  wires:
  u/1 -> DataWrite/1

== system elevator/PLCControllerSuite/__Logic/Task/Program/__Logic/OTE9/Instruction_Enable/Rung-condition-in is true/__CoreVarWrite ==
  u : Inport
  DataWrite : DataStoreWrite  DataStoreName=xxx_PLC_VAR_MemoryGoUp
  wires:
  u/1 -> DataWrite/1

== system elevator/PLCControllerSuite/__Logic/Task/Program/__Logic/OTE9/RungInOverride/ForceRungInFalseRead/__CoreLabelRead ==
  DataRead : DataStoreRead  DataStoreName=x_PLCLabel__s4_3653__Force_RungIn_False
  Out1 : Outport  VectorParamsAs1DForOutWhenUnconnected=off
  wires:
  DataRead/1 -> Out1/1

== system elevator/PLCControllerSuite/__Logic/Task/Program/__Logic/SUB/RungInOverride/ForceRungInFalseRead/__CoreLabelRead ==
  DataRead : DataStoreRead  DataStoreName=x_PLCLabel__s4_3653__Force_RungIn_False
  Out1 : Outport  VectorParamsAs1DForOutWhenUnconnected=off
  wires:
  DataRead/1 -> Out1/1

== system elevator/PLCControllerSuite/__Logic/Task/Program/__Logic/SUB/RungOutOverride/BlockEnableRead/__CoreLabelRead ==
  DataRead : DataStoreRead  DataStoreName=x_PLCLabel__s4_3653__Block_Enable
  Out1 : Outport  VectorParamsAs1DForOutWhenUnconnected=off
  wires:
  DataRead/1 -> Out1/1

== system elevator/PLCControllerSuite/__Logic/Task/Program/__Logic/SUB/RungOutOverride/VariableWriteEnableWrite/__CoreLabelWrite ==
  In1 : Inport
  DataWrite : DataStoreWrite  DataStoreName=x_PLCLabel__s4_3653__Variable_Write_Enable
  wires:
  In1/1 -> DataWrite/1

== system elevator/PLCControllerSuite/__Logic/Task/Program/__Logic/TON/Instruction_Enable/Initialize Function/VarWrite ==
  In1 : Inport
  __CoreVarWrite : Subsystem  Tag=CoreVarWriteBlock  DisableCoverage=on  TreatAsAtomicUnit=on  mask{PLCBlockType=CoreVarWrite}
      mask init:
      | slplc.callbacks.initCoreVariable(gcb, 'write');
      mask Help: web([docroot '/plccoder/ref/__corevarwrite' '.html']);
      mask DialogControl PLCBlockTitle Prompt: Core Variable Write
  wires:
  In1/1 -> __CoreVarWrite/1(u)

== system elevator/PLCControllerSuite/__Logic/Task/Program/__Logic/TON/Instruction_Enable/Initialize Function/VarWrite1 ==
  In1 : Inport
  __CoreVarWrite : Subsystem  Tag=CoreVarWriteBlock  DisableCoverage=on  TreatAsAtomicUnit=on  mask{PLCBlockType=CoreVarWrite}
      mask init:
      | slplc.callbacks.initCoreVariable(gcb, 'write');
      mask Help: web([docroot '/plccoder/ref/__corevarwrite' '.html']);
      mask DialogControl PLCBlockTitle Prompt: Core Variable Write
  wires:
  In1/1 -> __CoreVarWrite/1(u)

== system elevator/PLCControllerSuite/__Logic/Task/Program/__Logic/TON/Instruction_Enable/Initialize Function/VarWrite2 ==
  In1 : Inport
  __CoreVarWrite : Subsystem  Tag=CoreVarWriteBlock  DisableCoverage=on  TreatAsAtomicUnit=on  mask{PLCBlockType=CoreVarWrite}
      mask init:
      | slplc.callbacks.initCoreVariable(gcb, 'write');
      mask Help: web([docroot '/plccoder/ref/__corevarwrite' '.html']);
      mask DialogControl PLCBlockTitle Prompt: Core Variable Write
  wires:
  In1/1 -> __CoreVarWrite/1(u)

== system elevator/PLCControllerSuite/__Logic/Task/Program/__Logic/TON/Instruction_Enable/Initialize Function/VarWrite3 ==
  In1 : Inport
  __CoreVarWrite : Subsystem  Tag=CoreVarWriteBlock  DisableCoverage=on  TreatAsAtomicUnit=on  mask{PLCBlockType=CoreVarWrite}
      mask init:
      | slplc.callbacks.initCoreVariable(gcb, 'write');
      mask Help: web([docroot '/plccoder/ref/__corevarwrite' '.html']);
      mask DialogControl PLCBlockTitle Prompt: Core Variable Write
  wires:
  In1/1 -> __CoreVarWrite/1(u)

== system elevator/PLCControllerSuite/__Logic/Task/Program/__Logic/TON/RungInOverride/ForceRungInFalseRead/__CoreLabelRead ==
  DataRead : DataStoreRead  DataStoreName=x_PLCLabel__s4_3653__Force_RungIn_False
  Out1 : Outport  VectorParamsAs1DForOutWhenUnconnected=off
  wires:
  DataRead/1 -> Out1/1

== system elevator/PLCControllerSuite/__Logic/Task/Program/__Logic/XIC/RungInOverride/ForceRungInFalseRead/__CoreLabelRead ==
  DataRead : DataStoreRead  DataStoreName=x_PLCLabel__s4_3653__Force_RungIn_False
  Out1 : Outport  VectorParamsAs1DForOutWhenUnconnected=off
  wires:
  DataRead/1 -> Out1/1

== system elevator/PLCControllerSuite/__Logic/Task/Program/__Logic/XIC1/RungInOverride/ForceRungInFalseRead/__CoreLabelRead ==
  DataRead : DataStoreRead  DataStoreName=x_PLCLabel__s4_3653__Force_RungIn_False
  Out1 : Outport  VectorParamsAs1DForOutWhenUnconnected=off
  wires:
  DataRead/1 -> Out1/1

== system elevator/PLCControllerSuite/__Logic/Task/Program/__Logic/XIC10/RungInOverride/ForceRungInFalseRead/__CoreLabelRead ==
  DataRead : DataStoreRead  DataStoreName=x_PLCLabel__s4_3653__Force_RungIn_False
  Out1 : Outport  VectorParamsAs1DForOutWhenUnconnected=off
  wires:
  DataRead/1 -> Out1/1

== system elevator/PLCControllerSuite/__Logic/Task/Program/__Logic/XIC100/RungInOverride/ForceRungInFalseRead/__CoreLabelRead ==
  DataRead : DataStoreRead  DataStoreName=x_PLCLabel__s4_3653__Force_RungIn_False
  Out1 : Outport  VectorParamsAs1DForOutWhenUnconnected=off
  wires:
  DataRead/1 -> Out1/1

== system elevator/PLCControllerSuite/__Logic/Task/Program/__Logic/XIC101/RungInOverride/ForceRungInFalseRead/__CoreLabelRead ==
  DataRead : DataStoreRead  DataStoreName=x_PLCLabel__s4_3653__Force_RungIn_False
  Out1 : Outport  VectorParamsAs1DForOutWhenUnconnected=off
  wires:
  DataRead/1 -> Out1/1

== system elevator/PLCControllerSuite/__Logic/Task/Program/__Logic/XIC102/RungInOverride/ForceRungInFalseRead/__CoreLabelRead ==
  DataRead : DataStoreRead  DataStoreName=x_PLCLabel__s4_3653__Force_RungIn_False
  Out1 : Outport  VectorParamsAs1DForOutWhenUnconnected=off
  wires:
  DataRead/1 -> Out1/1

== system elevator/PLCControllerSuite/__Logic/Task/Program/__Logic/XIC103/RungInOverride/ForceRungInFalseRead/__CoreLabelRead ==
  DataRead : DataStoreRead  DataStoreName=x_PLCLabel__s4_3653__Force_RungIn_False
  Out1 : Outport  VectorParamsAs1DForOutWhenUnconnected=off
  wires:
  DataRead/1 -> Out1/1

== system elevator/PLCControllerSuite/__Logic/Task/Program/__Logic/XIC104/RungInOverride/ForceRungInFalseRead/__CoreLabelRead ==
  DataRead : DataStoreRead  DataStoreName=x_PLCLabel__s4_3653__Force_RungIn_False
  Out1 : Outport  VectorParamsAs1DForOutWhenUnconnected=off
  wires:
  DataRead/1 -> Out1/1

== system elevator/PLCControllerSuite/__Logic/Task/Program/__Logic/XIC105/RungInOverride/ForceRungInFalseRead/__CoreLabelRead ==
  DataRead : DataStoreRead  DataStoreName=x_PLCLabel__s4_3653__Force_RungIn_False
  Out1 : Outport  VectorParamsAs1DForOutWhenUnconnected=off
  wires:
  DataRead/1 -> Out1/1

== system elevator/PLCControllerSuite/__Logic/Task/Program/__Logic/XIC106/RungInOverride/ForceRungInFalseRead/__CoreLabelRead ==
  DataRead : DataStoreRead  DataStoreName=x_PLCLabel__s4_3653__Force_RungIn_False
  Out1 : Outport  VectorParamsAs1DForOutWhenUnconnected=off
  wires:
  DataRead/1 -> Out1/1

== system elevator/PLCControllerSuite/__Logic/Task/Program/__Logic/XIC107/RungInOverride/ForceRungInFalseRead/__CoreLabelRead ==
  DataRead : DataStoreRead  DataStoreName=x_PLCLabel__s4_3653__Force_RungIn_False
  Out1 : Outport  VectorParamsAs1DForOutWhenUnconnected=off
  wires:
  DataRead/1 -> Out1/1

== system elevator/PLCControllerSuite/__Logic/Task/Program/__Logic/XIC108/RungInOverride/ForceRungInFalseRead/__CoreLabelRead ==
  DataRead : DataStoreRead  DataStoreName=x_PLCLabel__s4_3653__Force_RungIn_False
  Out1 : Outport  VectorParamsAs1DForOutWhenUnconnected=off
  wires:
  DataRead/1 -> Out1/1

== system elevator/PLCControllerSuite/__Logic/Task/Program/__Logic/XIC109/RungInOverride/ForceRungInFalseRead/__CoreLabelRead ==
  DataRead : DataStoreRead  DataStoreName=x_PLCLabel__s4_3653__Force_RungIn_False
  Out1 : Outport  VectorParamsAs1DForOutWhenUnconnected=off
  wires:
  DataRead/1 -> Out1/1

== system elevator/PLCControllerSuite/__Logic/Task/Program/__Logic/XIC11/RungInOverride/ForceRungInFalseRead/__CoreLabelRead ==
  DataRead : DataStoreRead  DataStoreName=x_PLCLabel__s4_3653__Force_RungIn_False
  Out1 : Outport  VectorParamsAs1DForOutWhenUnconnected=off
  wires:
  DataRead/1 -> Out1/1

== system elevator/PLCControllerSuite/__Logic/Task/Program/__Logic/XIC110/RungInOverride/ForceRungInFalseRead/__CoreLabelRead ==
  DataRead : DataStoreRead  DataStoreName=x_PLCLabel__s4_3653__Force_RungIn_False
  Out1 : Outport  VectorParamsAs1DForOutWhenUnconnected=off
  wires:
  DataRead/1 -> Out1/1

== system elevator/PLCControllerSuite/__Logic/Task/Program/__Logic/XIC111/RungInOverride/ForceRungInFalseRead/__CoreLabelRead ==
  DataRead : DataStoreRead  DataStoreName=x_PLCLabel__s4_3653__Force_RungIn_False
  Out1 : Outport  VectorParamsAs1DForOutWhenUnconnected=off
  wires:
  DataRead/1 -> Out1/1

== system elevator/PLCControllerSuite/__Logic/Task/Program/__Logic/XIC112/RungInOverride/ForceRungInFalseRead/__CoreLabelRead ==
  DataRead : DataStoreRead  DataStoreName=x_PLCLabel__s4_3653__Force_RungIn_False
  Out1 : Outport  VectorParamsAs1DForOutWhenUnconnected=off
  wires:
  DataRead/1 -> Out1/1

== system elevator/PLCControllerSuite/__Logic/Task/Program/__Logic/XIC113/RungInOverride/ForceRungInFalseRead/__CoreLabelRead ==
  DataRead : DataStoreRead  DataStoreName=x_PLCLabel__s4_3653__Force_RungIn_False
  Out1 : Outport  VectorParamsAs1DForOutWhenUnconnected=off
  wires:
  DataRead/1 -> Out1/1

== system elevator/PLCControllerSuite/__Logic/Task/Program/__Logic/XIC114/RungInOverride/ForceRungInFalseRead/__CoreLabelRead ==
  DataRead : DataStoreRead  DataStoreName=x_PLCLabel__s4_3653__Force_RungIn_False
  Out1 : Outport  VectorParamsAs1DForOutWhenUnconnected=off
  wires:
  DataRead/1 -> Out1/1

== system elevator/PLCControllerSuite/__Logic/Task/Program/__Logic/XIC115/RungInOverride/ForceRungInFalseRead/__CoreLabelRead ==
  DataRead : DataStoreRead  DataStoreName=x_PLCLabel__s4_3653__Force_RungIn_False
  Out1 : Outport  VectorParamsAs1DForOutWhenUnconnected=off
  wires:
  DataRead/1 -> Out1/1

== system elevator/PLCControllerSuite/__Logic/Task/Program/__Logic/XIC116/RungInOverride/ForceRungInFalseRead/__CoreLabelRead ==
  DataRead : DataStoreRead  DataStoreName=x_PLCLabel__s4_3653__Force_RungIn_False
  Out1 : Outport  VectorParamsAs1DForOutWhenUnconnected=off
  wires:
  DataRead/1 -> Out1/1
